simulink model "Sqrt"  (R2017b)
settings: Solver=FixedStepDiscrete  StartTime=0.0  StopTime=10.0  FixedStep=0.200000  RelTol=1e-3
undefined symbols (not defined in the file): Newton, Raphson
settings Model: Creator=ktrinh  LastModifiedBy=hbourbou
settings DataIOCC: ExternalInput=input_struct  SaveFormat=StructureWithTime  SaveState=on
settings OptimizationCC: LifeSpan=inf
settings DebuggingCC: AlgebraicLoopMsg=error  SFUnexpectedBacktrackingDiag=warning  SFNoUnconditionalDefaultTransitionDiag=warning  SFExecutionAtInitializationDiag=none
settings HardwareCC: ProdBitPerSizeT=32  ProdBitPerPtrDiffT=32  ProdWordSize=32  ProdHWDeviceType=Specified
settings CodeAppCC: StateflowObjectComments=on
settings GRTTargetCC: TargetLangStandard=C89/C90 (ANSI)  GeneratePreprocessorConditionals=Disable all
settings ConfigComp: CovMetricSettings=dw  CovHtmlReporting=on  CovSaveCumulativeToWorkspaceVar=on  CovSaveSingleToWorkspaceVar=on  CovExternalEMLEnable=off

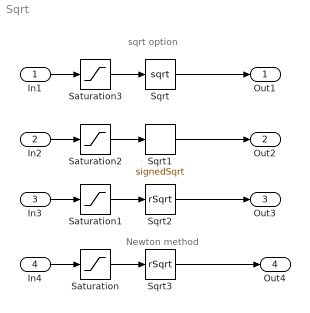
== system Sqrt ==
  note: sqrt option
  note: Newton method
  In1 : Inport  OutDataTypeStr=int32  PortDimensions=3
  In2 : Inport  Port=2  PortDimensions=3
  In3 : Inport  Port=3  PortDimensions=3
  In4 : Inport  Port=4  PortDimensions=3
  Saturation : Saturate  UpperLimit=inf  LowerLimit=0.1
  Saturation1 : Saturate  UpperLimit=inf  LowerLimit=0.1
  Saturation2 : Saturate  UpperLimit=inf  LowerLimit=0.1
  Saturation3 : Saturate  UpperLimit=300  LowerLimit=0.1
  Sqrt : Sqrt  SaturateOnIntegerOverflow=on
  Sqrt1 : Sqrt  Operator=signedSqrt  SaturateOnIntegerOverflow=on
  Sqrt2 : Sqrt  Operator=rSqrt  SaturateOnIntegerOverflow=on
  Sqrt3 : Sqrt  Operator=rSqrt  AlgorithmType=Newton-Raphson  SaturateOnIntegerOverflow=on
  Out1 : Outport
  Out2 : Outport  Port=2
  Out3 : Outport  Port=3
  Out4 : Outport  Port=4
  wires:
  In1/1 -> Saturation3/1
  Sqrt/1 -> Out1/1
  In2/1 -> Saturation2/1
  In3/1 -> Saturation1/1
  In4/1 -> Saturation/1
  Sqrt1/1 -> Out2/1
  Sqrt2/1 -> Out3/1
  Sqrt3/1 -> Out4/1
  Saturation/1 -> Sqrt3/1
  Saturation1/1 -> Sqrt2/1
  Saturation2/1 -> Sqrt1/1
  Saturation3/1 -> Sqrt/1
